simulink model "allmodes"  (Simulink 7.4)
settings: Solver=ode23tb  StartTime=0.0  StopTime=inf  MaxStep=1e-4  RelTol=1e-4
undefined symbols (not defined in the file): Ion, Lithium
libraries: powerlib x185, electricdrivelib x21, powerlib_extras x19, simulink x5
(part 3 of 7)

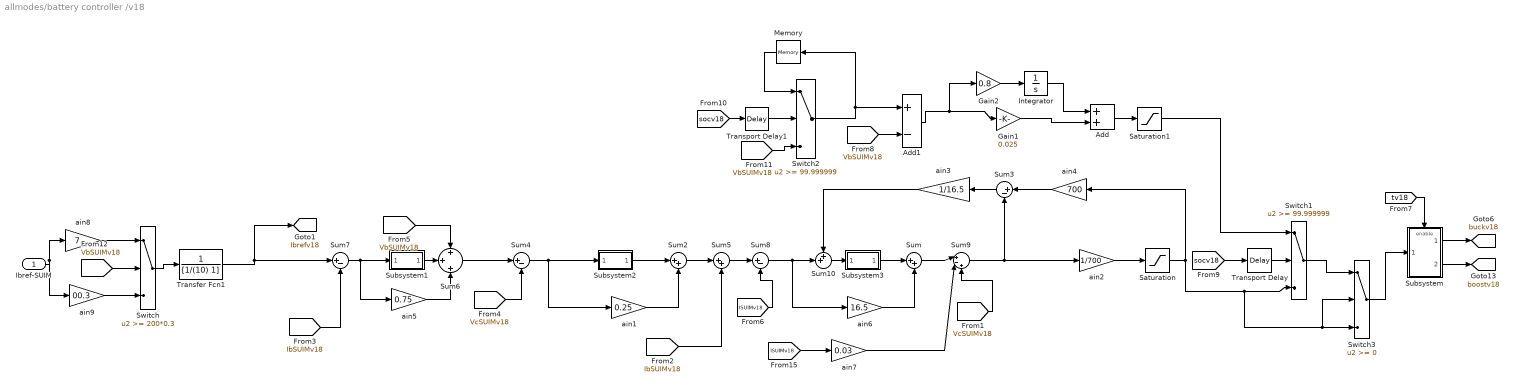
== system allmodes/battery controller /v18 ==
  Ibref-SUIM : Inport
  Add : Sum  OutDataType=fixdt(1, 16)  OutScaling=2^-10
  Add1 : Sum  Inputs=+-  OutDataType=fixdt(1, 16)  OutScaling=2^-10
  Gain1 : Gain  Gain=0.025  ParameterDataType=fixdt(1, 16)  ParameterScaling=2^0  OutDataType=fixdt(1, 16)  OutScaling=2^0
  Gain2 : Gain  Gain=0.8  ParameterDataType=fixdt(1, 16)  ParameterScaling=2^0  OutDataType=fixdt(1, 16)  OutScaling=2^0
  Integrator : Integrator
  Memory : Memory  X0=200
  Saturation : Saturate  UpperLimit=1  LowerLimit=-1  OutDataType=fixdt(1, 16)  OutScaling=2^0
  Saturation1 : Saturate  UpperLimit=1.01  LowerLimit=0.1  OutDataType=fixdt(1, 16)  OutScaling=2^0
  Subsystem : Subsystem
  Subsystem1 : Subsystem
  Subsystem2 : Subsystem
  Subsystem3 : Subsystem
  Sum : Sum  Inputs=|++  OutDataType=fixdt(1, 16)  OutScaling=2^0
  Sum10 : Sum  Inputs=++|  OutDataType=fixdt(1, 16)  OutScaling=2^0
  Sum2 : Sum  Inputs=|++  OutDataType=fixdt(1, 16)  OutScaling=2^0
  Sum{3..4,7..8} (4 alike) : Sum  Inputs=|+-  OutDataType=fixdt(1, 16)  OutScaling=2^0
  Sum5 : Sum  Inputs=|++  OutDataType=fixdt(1, 16)  OutScaling=2^0
  Sum6 : Sum  Inputs=+|+|+  OutDataType=fixdt(1, 16)  OutScaling=2^0
  Sum9 : Sum  Inputs=|+-+  OutDataType=fixdt(1, 16)  OutScaling=2^0
  Switch : Switch  Threshold=200*0.3  OutDataType=fixdt(1, 16)  OutScaling=2^0
  Switch1 : Switch  Threshold=99.999999  OutDataType=fixdt(1, 16)  OutScaling=2^0
  Switch2 : Switch  Threshold=99.999999  OutDataType=fixdt(1, 16)  OutScaling=2^0
  Switch3 : Switch  OutDataType=fixdt(1, 16)  OutScaling=2^0
  Transfer Fcn1 : TransferFcn  Numerator=1  Denominator=[1/(10) 1]
  Transport Delay : TransportDelay  DelayTime=2
  Transport Delay1 : TransportDelay  DelayTime=2
  ain1 : Gain  Gain=0.25  ParameterDataType=fixdt(1, 16)  ParameterScaling=2^0  OutDataType=fixdt(1, 16)  OutScaling=2^0
  ain2 : Gain  Gain=1/700  ParameterDataType=fixdt(1, 16)  ParameterScaling=2^0  OutDataType=fixdt(1, 16)  OutScaling=2^0
  ain3 : Gain  Gain=1/16.5  ParameterDataType=fixdt(1, 16)  ParameterScaling=2^0  OutDataType=fixdt(1, 16)  OutScaling=2^0
  ain4 : Gain  Gain=700  ParameterDataType=fixdt(1, 16)  ParameterScaling=2^0  OutDataType=fixdt(1, 16)  OutScaling=2^0
  ain5 : Gain  Gain=0.75  ParameterDataType=fixdt(1, 16)  ParameterScaling=2^0  OutDataType=fixdt(1, 16)  OutScaling=2^0
  ain6 : Gain  Gain=16.5  ParameterDataType=fixdt(1, 16)  ParameterScaling=2^0  OutDataType=fixdt(1, 16)  OutScaling=2^0
  ain7 : Gain  Gain=0.03  ParameterDataType=fixdt(1, 16)  ParameterScaling=2^0  OutDataType=fixdt(1, 16)  OutScaling=2^0
  ain8 : Gain  Gain=7  ParameterDataType=fixdt(1, 16)  ParameterScaling=2^0  OutDataType=fixdt(1, 16)  OutScaling=2^0
  ain9 : Gain  Gain=00.3  ParameterDataType=fixdt(1, 16)  ParameterScaling=2^0  OutDataType=fixdt(1, 16)  OutScaling=2^0
  tag scope: Ibrefv18=global, boostv18=global, buckv18=global
  wires:
  Ibref-SUIM/1 -> ain9/1, ain8/1
  Switch/1 -> Transfer Fcn1/1
  ain9/1 -> Switch/3
  ain8/1 -> Switch/1
  [VbSUIMv18] -> Switch/2
  Saturation1/1 -> Switch1/1
  Transport Delay/1 -> Switch1/2
  [socv18] -> Transport Delay/1
  Memory/1 -> Switch2/1
  Switch2/1 -> Memory/1, Add1/1
  Gain2/1 -> Integrator/1
  Integrator/1 -> Add/1
  Gain1/1 -> Add/2
  Add/1 -> Saturation1/1
  Transport Delay1/1 -> Switch2/2
  [socv18] -> Transport Delay1/1
  [VbSUIMv18] -> Switch2/3
  Add1/1 -> Gain2/1, Gain1/1
  [VbSUIMv18] -> Add1/2
  [tv18] -> Subsystem/Enable
  Sum4/1 -> ain1/1, Subsystem2/1(In1)
  ain2/1 -> Saturation/1
  Subsystem2/1(Out1) -> Sum2/1
  ain1/1 -> Sum2/2
  Saturation/1 -> ain4/1, Switch1/3, Switch3/3, Switch3/2
  ain4/1 -> Sum3/1
  Sum3/1 -> ain3/1
  Subsystem1/1(Out1) -> Sum6/2
  ain5/1 -> Sum6/3
  Sum7/1 -> ain5/1, Subsystem1/1(In1)
  Sum2/1 -> Sum5/1
  Sum5/1 -> Sum8/1
  Sum8/1 -> ain6/1, Sum10/2
  Subsystem3/1(Out1) -> Sum/1
  ain6/1 -> Sum/2
  Sum/1 -> Sum9/1
  Sum9/1 -> Sum3/2, ain2/1
  ain3/1 -> Sum10/1
  ain7/1 -> Sum9/2
  Sum6/1 -> Sum4/1
  Sum10/1 -> Subsystem3/1(In1)
  [VcSUIMv18] -> Sum4/2
  [VcSUIMv18] -> Sum9/3
  [IbSUIMv18] -> Sum7/2
  [IbSUIMv18] -> Sum5/2
  [VbSUIMv18] -> Sum6/1
  [ISUIMv18] -> ain7/1
  [ISUIMv18] -> Sum8/2
  Subsystem/2(Out2) -> [boostv18]
  Subsystem/1(Out1) -> [buckv18]
  Transfer Fcn1/1 -> [Ibrefv18], Sum7/1
  Switch1/1 -> Switch3/1
  Switch3/1 -> Subsystem/1(In1)

== system allmodes/battery controller /v19 ==
  Ibref-SUIM : Inport
  Add : Sum  OutDataType=fixdt(1, 16)  OutScaling=2^-10
  Add1 : Sum  Inputs=+-  OutDataType=fixdt(1, 16)  OutScaling=2^-10
  Gain1 : Gain  Gain=0.025  ParameterDataType=fixdt(1, 16)  ParameterScaling=2^0  OutDataType=fixdt(1, 16)  OutScaling=2^0
  Gain2 : Gain  Gain=0.8  ParameterDataType=fixdt(1, 16)  ParameterScaling=2^0  OutDataType=fixdt(1, 16)  OutScaling=2^0
  Integrator : Integrator
  Memory : Memory  X0=200
  Saturation : Saturate  UpperLimit=1  LowerLimit=-1  OutDataType=fixdt(1, 16)  OutScaling=2^0
  Saturation1 : Saturate  UpperLimit=1.01  LowerLimit=0.1  OutDataType=fixdt(1, 16)  OutScaling=2^0
  Subsystem : Subsystem
  Subsystem1 : Subsystem
  Subsystem2 : Subsystem
  Subsystem3 : Subsystem
  Sum : Sum  Inputs=|++  OutDataType=fixdt(1, 16)  OutScaling=2^0
  Sum10 : Sum  Inputs=++|  OutDataType=fixdt(1, 16)  OutScaling=2^0
  Sum2 : Sum  Inputs=|++  OutDataType=fixdt(1, 16)  OutScaling=2^0
  Sum{3..4,7..8} (4 alike) : Sum  Inputs=|+-  OutDataType=fixdt(1, 16)  OutScaling=2^0
  Sum5 : Sum  Inputs=|++  OutDataType=fixdt(1, 16)  OutScaling=2^0
  Sum6 : Sum  Inputs=+|+|+  OutDataType=fixdt(1, 16)  OutScaling=2^0
  Sum9 : Sum  Inputs=|+-+  OutDataType=fixdt(1, 16)  OutScaling=2^0
  Switch : Switch  Threshold=200*0.3  OutDataType=fixdt(1, 16)  OutScaling=2^0
  Switch1 : Switch  Threshold=99.999999  OutDataType=fixdt(1, 16)  OutScaling=2^0
  Switch2 : Switch  Threshold=99.999999  OutDataType=fixdt(1, 16)  OutScaling=2^0
  Switch3 : Switch  OutDataType=fixdt(1, 16)  OutScaling=2^0
  Transfer Fcn1 : TransferFcn  Numerator=1  Denominator=[1/(10) 1]
  Transport Delay : TransportDelay  DelayTime=2
  Transport Delay1 : TransportDelay  DelayTime=2
  ain1 : Gain  Gain=0.25  ParameterDataType=fixdt(1, 16)  ParameterScaling=2^0  OutDataType=fixdt(1, 16)  OutScaling=2^0
  ain2 : Gain  Gain=1/700  ParameterDataType=fixdt(1, 16)  ParameterScaling=2^0  OutDataType=fixdt(1, 16)  OutScaling=2^0
  ain3 : Gain  Gain=1/16.5  ParameterDataType=fixdt(1, 16)  ParameterScaling=2^0  OutDataType=fixdt(1, 16)  OutScaling=2^0
  ain4 : Gain  Gain=700  ParameterDataType=fixdt(1, 16)  ParameterScaling=2^0  OutDataType=fixdt(1, 16)  OutScaling=2^0
  ain5 : Gain  Gain=0.75  ParameterDataType=fixdt(1, 16)  ParameterScaling=2^0  OutDataType=fixdt(1, 16)  OutScaling=2^0
  ain6 : Gain  Gain=16.5  ParameterDataType=fixdt(1, 16)  ParameterScaling=2^0  OutDataType=fixdt(1, 16)  OutScaling=2^0
  ain7 : Gain  Gain=0.03  ParameterDataType=fixdt(1, 16)  ParameterScaling=2^0  OutDataType=fixdt(1, 16)  OutScaling=2^0
  ain8 : Gain  Gain=7  ParameterDataType=fixdt(1, 16)  ParameterScaling=2^0  OutDataType=fixdt(1, 16)  OutScaling=2^0
  ain9 : Gain  Gain=0.3  ParameterDataType=fixdt(1, 16)  ParameterScaling=2^0  OutDataType=fixdt(1, 16)  OutScaling=2^0
  tag scope: Ibrefv19=global, boostv19=global, buckv19=global
  wires:
  Ibref-SUIM/1 -> ain9/1, ain8/1
  Switch/1 -> Transfer Fcn1/1
  ain9/1 -> Switch/3
  ain8/1 -> Switch/1
  [VbSUIMv19] -> Switch/2
  Saturation1/1 -> Switch1/1
  Transport Delay/1 -> Switch1/2
  [socv19] -> Transport Delay/1
  Memory/1 -> Switch2/1
  Switch2/1 -> Memory/1, Add1/1
  Gain2/1 -> Integrator/1
  Integrator/1 -> Add/1
  Gain1/1 -> Add/2
  Add/1 -> Saturation1/1
  Transport Delay1/1 -> Switch2/2
  [socv19] -> Transport Delay1/1
  [VbSUIMv19] -> Switch2/3
  Add1/1 -> Gain2/1, Gain1/1
  [VbSUIMv19] -> Add1/2
  [tv19] -> Subsystem/Enable
  Sum4/1 -> ain1/1, Subsystem2/1(In1)
  ain2/1 -> Saturation/1
  Subsystem2/1(Out1) -> Sum2/1
  ain1/1 -> Sum2/2
  Saturation/1 -> ain4/1, Switch1/3, Switch3/3, Switch3/2
  ain4/1 -> Sum3/1
  Sum3/1 -> ain3/1
  Subsystem1/1(Out1) -> Sum6/2
  ain5/1 -> Sum6/3
  Sum7/1 -> ain5/1, Subsystem1/1(In1)
  Sum2/1 -> Sum5/1
  Sum5/1 -> Sum8/1
  Sum8/1 -> ain6/1, Sum10/2
  Subsystem3/1(Out1) -> Sum/1
  ain6/1 -> Sum/2
  Sum/1 -> Sum9/1
  Sum9/1 -> Sum3/2, ain2/1
  ain3/1 -> Sum10/1
  ain7/1 -> Sum9/2
  Sum6/1 -> Sum4/1
  Sum10/1 -> Subsystem3/1(In1)
  [VcSUIMv19] -> Sum4/2
  [VcSUIMv19] -> Sum9/3
  [IbSUIMv19] -> Sum7/2
  [IbSUIMv19] -> Sum5/2
  [VbSUIMv19] -> Sum6/1
  [ISUIMv19] -> ain7/1
  [ISUIMv19] -> Sum8/2
  Subsystem/2(Out2) -> [boostv19]
  Subsystem/1(Out1) -> [buckv19]
  Transfer Fcn1/1 -> [Ibrefv19], Sum7/1
  Switch1/1 -> Switch3/1
  Switch3/1 -> Subsystem/1(In1)

== system allmodes/battery controller /v2 ==
  Ibref-v2 : Inport
  Add : Sum  OutDataType=fixdt(1, 16)  OutScaling=2^-10
  Add1 : Sum  Inputs=+-  OutDataType=fixdt(1, 16)  OutScaling=2^-10
  Gain1 : Gain  Gain=0.025  ParameterDataType=fixdt(1, 16)  ParameterScaling=2^0  OutDataType=fixdt(1, 16)  OutScaling=2^0
  Gain2 : Gain  Gain=0.8  ParameterDataType=fixdt(1, 16)  ParameterScaling=2^0  OutDataType=fixdt(1, 16)  OutScaling=2^0
  Integrator : Integrator
  Memory : Memory  X0=200
  Saturation : Saturate  UpperLimit=1  LowerLimit=-1  OutDataType=fixdt(1, 16)  OutScaling=2^0
  Saturation1 : Saturate  UpperLimit=1.01  LowerLimit=0.1  OutDataType=fixdt(1, 16)  OutScaling=2^0
  Subsystem : Subsystem
  Subsystem1 : Subsystem
  Subsystem2 : Subsystem
  Subsystem3 : Subsystem
  Sum : Sum  Inputs=|++  OutDataType=fixdt(1, 16)  OutScaling=2^0
  Sum10 : Sum  Inputs=++|  OutDataType=fixdt(1, 16)  OutScaling=2^0
  Sum2 : Sum  Inputs=|++  OutDataType=fixdt(1, 16)  OutScaling=2^0
  Sum{3..4,7..8} (4 alike) : Sum  Inputs=|+-  OutDataType=fixdt(1, 16)  OutScaling=2^0
  Sum5 : Sum  Inputs=|++  OutDataType=fixdt(1, 16)  OutScaling=2^0
  Sum6 : Sum  Inputs=+|+|+  OutDataType=fixdt(1, 16)  OutScaling=2^0
  Sum9 : Sum  Inputs=|+-+  OutDataType=fixdt(1, 16)  OutScaling=2^0
  Switch : Switch  Threshold=200*0.3  OutDataType=fixdt(1, 16)  OutScaling=2^0
  Switch1 : Switch  Threshold=99.999999  OutDataType=fixdt(1, 16)  OutScaling=2^0
  Switch2 : Switch  Threshold=99.999999  OutDataType=fixdt(1, 16)  OutScaling=2^0
  Switch3 : Switch  OutDataType=fixdt(1, 16)  OutScaling=2^0
  Transfer Fcn1 : TransferFcn  Numerator=1  Denominator=[1/(10) 1]
  Transport Delay : TransportDelay  DelayTime=2
  Transport Delay1 : TransportDelay  DelayTime=2
  ain1 : Gain  Gain=0.25  ParameterDataType=fixdt(1, 16)  ParameterScaling=2^0  OutDataType=fixdt(1, 16)  OutScaling=2^0
  ain2 : Gain  Gain=1/700  ParameterDataType=fixdt(1, 16)  ParameterScaling=2^0  OutDataType=fixdt(1, 16)  OutScaling=2^0
  ain3 : Gain  Gain=1/16.5  ParameterDataType=fixdt(1, 16)  ParameterScaling=2^0  OutDataType=fixdt(1, 16)  OutScaling=2^0
  ain4 : Gain  Gain=700  ParameterDataType=fixdt(1, 16)  ParameterScaling=2^0  OutDataType=fixdt(1, 16)  OutScaling=2^0
  ain5 : Gain  Gain=0.75  ParameterDataType=fixdt(1, 16)  ParameterScaling=2^0  OutDataType=fixdt(1, 16)  OutScaling=2^0
  ain6 : Gain  Gain=16.5  ParameterDataType=fixdt(1, 16)  ParameterScaling=2^0  OutDataType=fixdt(1, 16)  OutScaling=2^0
  ain7 : Gain  Gain=0.03  ParameterDataType=fixdt(1, 16)  ParameterScaling=2^0  OutDataType=fixdt(1, 16)  OutScaling=2^0
  ain8 : Gain  Gain=7  ParameterDataType=fixdt(1, 16)  ParameterScaling=2^0  OutDataType=fixdt(1, 16)  OutScaling=2^0
  ain9 : Gain  Gain=0.3  ParameterDataType=fixdt(1, 16)  ParameterScaling=2^0  OutDataType=fixdt(1, 16)  OutScaling=2^0
  tag scope: Ibrefv2=global, boostv2=global, buckv2=global
  wires:
  Sum4/1 -> ain1/1, Subsystem2/1(In1)
  ain2/1 -> Saturation/1
  Subsystem2/1(Out1) -> Sum2/1
  ain1/1 -> Sum2/2
  Saturation/1 -> ain4/1, Switch1/3, Switch3/2, Switch3/3
  ain4/1 -> Sum3/1
  Sum3/1 -> ain3/1
  Subsystem1/1(Out1) -> Sum6/2
  ain5/1 -> Sum6/3
  Sum7/1 -> ain5/1, Subsystem1/1(In1)
  Sum2/1 -> Sum5/1
  Sum5/1 -> Sum8/1
  Sum8/1 -> ain6/1, Sum10/2
  Subsystem3/1(Out1) -> Sum/1
  ain6/1 -> Sum/2
  Sum/1 -> Sum9/1
  Sum9/1 -> Sum3/2, ain2/1
  ain3/1 -> Sum10/1
  ain7/1 -> Sum9/2
  Sum6/1 -> Sum4/1
  Sum10/1 -> Subsystem3/1(In1)
  [VcSUIMv2] -> Sum4/2
  [VcSUIMv2] -> Sum9/3
  [IbSUIMv2] -> Sum7/2
  [IbSUIMv2] -> Sum5/2
  [VbSUIMv2] -> Sum6/1
  [ISUIMv2] -> ain7/1
  [ISUIMv2] -> Sum8/2
  Subsystem/2(Out2) -> [boostv2]
  Subsystem/1(Out1) -> [buckv2]
  Transfer Fcn1/1 -> [Ibrefv2], Sum7/1
  [tv2] -> Subsystem/Enable
  [VbSUIMv2] -> Switch/2
  ain8/1 -> Switch/1
  ain9/1 -> Switch/3
  Ibref-v2/1 -> ain8/1, ain9/1
  Switch/1 -> Transfer Fcn1/1
  [VbSUIMv2] -> Add1/2
  Add1/1 -> Gain1/1, Gain2/1
  [VbSUIMv2] -> Switch2/3
  [socv2] -> Transport Delay1/1
  Transport Delay1/1 -> Switch2/2
  Add/1 -> Saturation1/1
  Gain1/1 -> Add/2
  Integrator/1 -> Add/1
  Gain2/1 -> Integrator/1
  Switch2/1 -> Add1/1, Memory/1
  Memory/1 -> Switch2/1
  Saturation1/1 -> Switch1/1
  Transport Delay/1 -> Switch1/2
  [socv2] -> Transport Delay/1
  Switch1/1 -> Switch3/1
  Switch3/1 -> Subsystem/1(In1)

== system allmodes/battery controller /v20 ==
  Ibref-v2 : Inport
  Add : Sum  OutDataType=fixdt(1, 16)  OutScaling=2^-10
  Add1 : Sum  Inputs=+-  OutDataType=fixdt(1, 16)  OutScaling=2^-10
  Gain1 : Gain  Gain=0.025  ParameterDataType=fixdt(1, 16)  ParameterScaling=2^0  OutDataType=fixdt(1, 16)  OutScaling=2^0
  Gain2 : Gain  Gain=0.8  ParameterDataType=fixdt(1, 16)  ParameterScaling=2^0  OutDataType=fixdt(1, 16)  OutScaling=2^0
  Integrator : Integrator
  Memory : Memory  X0=200
  Saturation : Saturate  UpperLimit=1  LowerLimit=-1  OutDataType=fixdt(1, 16)  OutScaling=2^0
  Saturation1 : Saturate  UpperLimit=1.01  LowerLimit=0.1  OutDataType=fixdt(1, 16)  OutScaling=2^0
  Subsystem : Subsystem
  Subsystem1 : Subsystem
  Subsystem2 : Subsystem
  Subsystem3 : Subsystem
  Sum : Sum  Inputs=|++  OutDataType=fixdt(1, 16)  OutScaling=2^0
  Sum10 : Sum  Inputs=++|  OutDataType=fixdt(1, 16)  OutScaling=2^0
  Sum2 : Sum  Inputs=|++  OutDataType=fixdt(1, 16)  OutScaling=2^0
  Sum{3..4,7..8} (4 alike) : Sum  Inputs=|+-  OutDataType=fixdt(1, 16)  OutScaling=2^0
  Sum5 : Sum  Inputs=|++  OutDataType=fixdt(1, 16)  OutScaling=2^0
  Sum6 : Sum  Inputs=+|+|+  OutDataType=fixdt(1, 16)  OutScaling=2^0
  Sum9 : Sum  Inputs=|+-+  OutDataType=fixdt(1, 16)  OutScaling=2^0
  Switch : Switch  Threshold=200*0.3  OutDataType=fixdt(1, 16)  OutScaling=2^0
  Switch1 : Switch  Threshold=99.999999  OutDataType=fixdt(1, 16)  OutScaling=2^0
  Switch2 : Switch  Threshold=99.999999  OutDataType=fixdt(1, 16)  OutScaling=2^0
  Switch3 : Switch  OutDataType=fixdt(1, 16)  OutScaling=2^0
  Transfer Fcn1 : TransferFcn  Numerator=1  Denominator=[1/(10) 1]
  Transport Delay : TransportDelay  DelayTime=2
  Transport Delay1 : TransportDelay  DelayTime=2
  ain1 : Gain  Gain=0.25  ParameterDataType=fixdt(1, 16)  ParameterScaling=2^0  OutDataType=fixdt(1, 16)  OutScaling=2^0
  ain2 : Gain  Gain=1/700  ParameterDataType=fixdt(1, 16)  ParameterScaling=2^0  OutDataType=fixdt(1, 16)  OutScaling=2^0
  ain3 : Gain  Gain=1/16.5  ParameterDataType=fixdt(1, 16)  ParameterScaling=2^0  OutDataType=fixdt(1, 16)  OutScaling=2^0
  ain4 : Gain  Gain=700  ParameterDataType=fixdt(1, 16)  ParameterScaling=2^0  OutDataType=fixdt(1, 16)  OutScaling=2^0
  ain5 : Gain  Gain=0.75  ParameterDataType=fixdt(1, 16)  ParameterScaling=2^0  OutDataType=fixdt(1, 16)  OutScaling=2^0
  ain6 : Gain  Gain=16.5  ParameterDataType=fixdt(1, 16)  ParameterScaling=2^0  OutDataType=fixdt(1, 16)  OutScaling=2^0
  ain7 : Gain  Gain=0.03  ParameterDataType=fixdt(1, 16)  ParameterScaling=2^0  OutDataType=fixdt(1, 16)  OutScaling=2^0
  ain8 : Gain  Gain=7  ParameterDataType=fixdt(1, 16)  ParameterScaling=2^0  OutDataType=fixdt(1, 16)  OutScaling=2^0
  ain9 : Gain  Gain=0.3  ParameterDataType=fixdt(1, 16)  ParameterScaling=2^0  OutDataType=fixdt(1, 16)  OutScaling=2^0
  tag scope: Ibrefv20=global, boostv20=global, buckv20=global
  wires:
  [socv20] -> Transport Delay/1
  Transport Delay/1 -> Switch1/2
  Saturation1/1 -> Switch1/1
  Memory/1 -> Switch2/1
  Switch2/1 -> Memory/1, Add1/1
  Gain2/1 -> Integrator/1
  Integrator/1 -> Add/1
  Gain1/1 -> Add/2
  Add/1 -> Saturation1/1
  Transport Delay1/1 -> Switch2/2
  [socv20] -> Transport Delay1/1
  [VbSUIMv20] -> Switch2/3
  Add1/1 -> Gain2/1, Gain1/1
  [VbSUIMv20] -> Add1/2
  Switch/1 -> Transfer Fcn1/1
  Ibref-v2/1 -> ain9/1, ain8/1
  ain9/1 -> Switch/3
  ain8/1 -> Switch/1
  [VbSUIMv20] -> Switch/2
  [tv20] -> Subsystem/Enable
  Transfer Fcn1/1 -> Sum7/1, [Ibrefv20]
  Subsystem/1(Out1) -> [buckv20]
  Subsystem/2(Out2) -> [boostv20]
  [ISUIMv20] -> Sum8/2
  [ISUIMv20] -> ain7/1
  [VbSUIMv20] -> Sum6/1
  [IbSUIMv20] -> Sum5/2
  [IbSUIMv20] -> Sum7/2
  [VcSUIMv20] -> Sum9/3
  [VcSUIMv20] -> Sum4/2
  Sum10/1 -> Subsystem3/1(In1)
  Sum6/1 -> Sum4/1
  ain7/1 -> Sum9/2
  ain3/1 -> Sum10/1
  Sum9/1 -> ain2/1, Sum3/2
  Sum/1 -> Sum9/1
  ain6/1 -> Sum/2
  Subsystem3/1(Out1) -> Sum/1
  Sum8/1 -> Sum10/2, ain6/1
  Sum5/1 -> Sum8/1
  Sum2/1 -> Sum5/1
  Sum7/1 -> Subsystem1/1(In1), ain5/1
  ain5/1 -> Sum6/3
  Subsystem1/1(Out1) -> Sum6/2
  Sum3/1 -> ain3/1
  ain4/1 -> Sum3/1
  Saturation/1 -> ain4/1, Switch1/3, Switch3/3, Switch3/2
  ain1/1 -> Sum2/2
  Subsystem2/1(Out1) -> Sum2/1
  ain2/1 -> Saturation/1
  Sum4/1 -> Subsystem2/1(In1), ain1/1
  Switch1/1 -> Switch3/1
  Switch3/1 -> Subsystem/1(In1)

== system allmodes/battery controller /v3 ==
  Ibref-v2 : Inport
  Add : Sum  OutDataType=fixdt(1, 16)  OutScaling=2^-10
  Add1 : Sum  Inputs=+-  OutDataType=fixdt(1, 16)  OutScaling=2^-10
  Gain1 : Gain  Gain=0.025  ParameterDataType=fixdt(1, 16)  ParameterScaling=2^0  OutDataType=fixdt(1, 16)  OutScaling=2^0
  Gain2 : Gain  Gain=0.8  ParameterDataType=fixdt(1, 16)  ParameterScaling=2^0  OutDataType=fixdt(1, 16)  OutScaling=2^0
  Integrator : Integrator
  Memory : Memory  X0=200
  Saturation : Saturate  UpperLimit=1  LowerLimit=-1  OutDataType=fixdt(1, 16)  OutScaling=2^0
  Saturation1 : Saturate  UpperLimit=1.01  LowerLimit=0.1  OutDataType=fixdt(1, 16)  OutScaling=2^0
  Subsystem : Subsystem
  Subsystem1 : Subsystem
  Subsystem2 : Subsystem
  Subsystem3 : Subsystem
  Sum : Sum  Inputs=|++  OutDataType=fixdt(1, 16)  OutScaling=2^0
  Sum10 : Sum  Inputs=++|  OutDataType=fixdt(1, 16)  OutScaling=2^0
  Sum2 : Sum  Inputs=|++  OutDataType=fixdt(1, 16)  OutScaling=2^0
  Sum{3..4,7..8} (4 alike) : Sum  Inputs=|+-  OutDataType=fixdt(1, 16)  OutScaling=2^0
  Sum5 : Sum  Inputs=|++  OutDataType=fixdt(1, 16)  OutScaling=2^0
  Sum6 : Sum  Inputs=+|+|+  OutDataType=fixdt(1, 16)  OutScaling=2^0
  Sum9 : Sum  Inputs=|+-+  OutDataType=fixdt(1, 16)  OutScaling=2^0
  Switch : Switch  Threshold=200*0.3  OutDataType=fixdt(1, 16)  OutScaling=2^0
  Switch1 : Switch  Threshold=99.999999  OutDataType=fixdt(1, 16)  OutScaling=2^0
  Switch2 : Switch  Threshold=99.999999  OutDataType=fixdt(1, 16)  OutScaling=2^0
  Switch3 : Switch  OutDataType=fixdt(1, 16)  OutScaling=2^0
  Transfer Fcn1 : TransferFcn  Numerator=1  Denominator=[1/(10) 1]
  Transport Delay : TransportDelay  DelayTime=2
  Transport Delay1 : TransportDelay  DelayTime=2
  ain1 : Gain  Gain=0.25  ParameterDataType=fixdt(1, 16)  ParameterScaling=2^0  OutDataType=fixdt(1, 16)  OutScaling=2^0
  ain2 : Gain  Gain=1/700  ParameterDataType=fixdt(1, 16)  ParameterScaling=2^0  OutDataType=fixdt(1, 16)  OutScaling=2^0
  ain3 : Gain  Gain=1/16.5  ParameterDataType=fixdt(1, 16)  ParameterScaling=2^0  OutDataType=fixdt(1, 16)  OutScaling=2^0
  ain4 : Gain  Gain=700  ParameterDataType=fixdt(1, 16)  ParameterScaling=2^0  OutDataType=fixdt(1, 16)  OutScaling=2^0
  ain5 : Gain  Gain=0.75  ParameterDataType=fixdt(1, 16)  ParameterScaling=2^0  OutDataType=fixdt(1, 16)  OutScaling=2^0
  ain6 : Gain  Gain=16.5  ParameterDataType=fixdt(1, 16)  ParameterScaling=2^0  OutDataType=fixdt(1, 16)  OutScaling=2^0
  ain7 : Gain  Gain=0.03  ParameterDataType=fixdt(1, 16)  ParameterScaling=2^0  OutDataType=fixdt(1, 16)  OutScaling=2^0
  ain8 : Gain  Gain=7  ParameterDataType=fixdt(1, 16)  ParameterScaling=2^0  OutDataType=fixdt(1, 16)  OutScaling=2^0
  ain9 : Gain  Gain=0.3  ParameterDataType=fixdt(1, 16)  ParameterScaling=2^0  OutDataType=fixdt(1, 16)  OutScaling=2^0
  tag scope: Ibrefv3=global, boostv3=global, buckv3=global
  wires:
  [socv3] -> Transport Delay/1
  Transport Delay/1 -> Switch1/2
  Saturation1/1 -> Switch1/1
  Memory/1 -> Switch2/1
  Switch2/1 -> Memory/1, Add1/1
  Gain2/1 -> Integrator/1
  Integrator/1 -> Add/1
  Gain1/1 -> Add/2
  Add/1 -> Saturation1/1
  Transport Delay1/1 -> Switch2/2
  [socv3] -> Transport Delay1/1
  [VbSUIMv3] -> Switch2/3
  Add1/1 -> Gain2/1, Gain1/1
  [VbSUIMv3] -> Add1/2
  Switch/1 -> Transfer Fcn1/1
  Ibref-v2/1 -> ain9/1, ain8/1
  ain9/1 -> Switch/3
  ain8/1 -> Switch/1
  [VbSUIMv3] -> Switch/2
  [tv3] -> Subsystem/Enable
  Transfer Fcn1/1 -> Sum7/1, [Ibrefv3]
  Subsystem/1(Out1) -> [buckv3]
  Subsystem/2(Out2) -> [boostv3]
  [ISUIMv3] -> Sum8/2
  [ISUIMv3] -> ain7/1
  [VbSUIMv3] -> Sum6/1
  [IbSUIMv3] -> Sum5/2
  [IbSUIMv3] -> Sum7/2
  [VcSUIMv3] -> Sum9/3
  [VcSUIMv3] -> Sum4/2
  Sum10/1 -> Subsystem3/1(In1)
  Sum6/1 -> Sum4/1
  ain7/1 -> Sum9/2
  ain3/1 -> Sum10/1
  Sum9/1 -> ain2/1, Sum3/2
  Sum/1 -> Sum9/1
  ain6/1 -> Sum/2
  Subsystem3/1(Out1) -> Sum/1
  Sum8/1 -> Sum10/2, ain6/1
  Sum5/1 -> Sum8/1
  Sum2/1 -> Sum5/1
  Sum7/1 -> Subsystem1/1(In1), ain5/1
  ain5/1 -> Sum6/3
  Subsystem1/1(Out1) -> Sum6/2
  Sum3/1 -> ain3/1
  ain4/1 -> Sum3/1
  Saturation/1 -> ain4/1, Switch1/3, Switch3/2, Switch3/3
  ain1/1 -> Sum2/2
  Subsystem2/1(Out1) -> Sum2/1
  ain2/1 -> Saturation/1
  Sum4/1 -> Subsystem2/1(In1), ain1/1
  Switch1/1 -> Switch3/1
  Switch3/1 -> Subsystem/1(In1)

== system allmodes/battery controller /v4 ==
  Ibref-v2 : Inport
  Add : Sum  OutDataType=fixdt(1, 16)  OutScaling=2^-10
  Add1 : Sum  Inputs=+-  OutDataType=fixdt(1, 16)  OutScaling=2^-10
  Gain1 : Gain  Gain=0.025  ParameterDataType=fixdt(1, 16)  ParameterScaling=2^0  OutDataType=fixdt(1, 16)  OutScaling=2^0
  Gain2 : Gain  Gain=0.8  ParameterDataType=fixdt(1, 16)  ParameterScaling=2^0  OutDataType=fixdt(1, 16)  OutScaling=2^0
  Integrator : Integrator
  Memory : Memory  X0=200
  Saturation : Saturate  UpperLimit=1  LowerLimit=-1  OutDataType=fixdt(1, 16)  OutScaling=2^0
  Saturation1 : Saturate  UpperLimit=1.01  LowerLimit=0.1  OutDataType=fixdt(1, 16)  OutScaling=2^0
  Subsystem : Subsystem
  Subsystem1 : Subsystem
  Subsystem2 : Subsystem
  Subsystem3 : Subsystem
  Sum : Sum  Inputs=|++  OutDataType=fixdt(1, 16)  OutScaling=2^0
  Sum10 : Sum  Inputs=++|  OutDataType=fixdt(1, 16)  OutScaling=2^0
  Sum2 : Sum  Inputs=|++  OutDataType=fixdt(1, 16)  OutScaling=2^0
  Sum{3..4,7..8} (4 alike) : Sum  Inputs=|+-  OutDataType=fixdt(1, 16)  OutScaling=2^0
  Sum5 : Sum  Inputs=|++  OutDataType=fixdt(1, 16)  OutScaling=2^0
  Sum6 : Sum  Inputs=+|+|+  OutDataType=fixdt(1, 16)  OutScaling=2^0
  Sum9 : Sum  Inputs=|+-+  OutDataType=fixdt(1, 16)  OutScaling=2^0
  Switch : Switch  Threshold=200*0.3  OutDataType=fixdt(1, 16)  OutScaling=2^0
  Switch1 : Switch  Threshold=99.999999  OutDataType=fixdt(1, 16)  OutScaling=2^0
  Switch2 : Switch  Threshold=99.999999  OutDataType=fixdt(1, 16)  OutScaling=2^0
  Switch3 : Switch  OutDataType=fixdt(1, 16)  OutScaling=2^0
  Transfer Fcn1 : TransferFcn  Numerator=1  Denominator=[1/(10) 1]
  Transport Delay : TransportDelay  DelayTime=2
  Transport Delay1 : TransportDelay  DelayTime=2
  ain1 : Gain  Gain=0.25  ParameterDataType=fixdt(1, 16)  ParameterScaling=2^0  OutDataType=fixdt(1, 16)  OutScaling=2^0
  ain2 : Gain  Gain=1/700  ParameterDataType=fixdt(1, 16)  ParameterScaling=2^0  OutDataType=fixdt(1, 16)  OutScaling=2^0
  ain3 : Gain  Gain=1/16.5  ParameterDataType=fixdt(1, 16)  ParameterScaling=2^0  OutDataType=fixdt(1, 16)  OutScaling=2^0
  ain4 : Gain  Gain=700  ParameterDataType=fixdt(1, 16)  ParameterScaling=2^0  OutDataType=fixdt(1, 16)  OutScaling=2^0
  ain5 : Gain  Gain=0.75  ParameterDataType=fixdt(1, 16)  ParameterScaling=2^0  OutDataType=fixdt(1, 16)  OutScaling=2^0
  ain6 : Gain  Gain=16.5  ParameterDataType=fixdt(1, 16)  ParameterScaling=2^0  OutDataType=fixdt(1, 16)  OutScaling=2^0
  ain7 : Gain  Gain=0.03  ParameterDataType=fixdt(1, 16)  ParameterScaling=2^0  OutDataType=fixdt(1, 16)  OutScaling=2^0
  ain8 : Gain  Gain=7  ParameterDataType=fixdt(1, 16)  ParameterScaling=2^0  OutDataType=fixdt(1, 16)  OutScaling=2^0
  ain9 : Gain  Gain=0.3  ParameterDataType=fixdt(1, 16)  ParameterScaling=2^0  OutDataType=fixdt(1, 16)  OutScaling=2^0
  tag scope: Ibrefv4=global, boostv4=global, buckv4=global
  wires:
  Sum4/1 -> ain1/1, Subsystem2/1(In1)
  ain2/1 -> Saturation/1
  Subsystem2/1(Out1) -> Sum2/1
  ain1/1 -> Sum2/2
  Saturation/1 -> ain4/1, Switch1/3, Switch3/2, Switch3/3
  ain4/1 -> Sum3/1
  Sum3/1 -> ain3/1
  Subsystem1/1(Out1) -> Sum6/2
  ain5/1 -> Sum6/3
  Sum7/1 -> ain5/1, Subsystem1/1(In1)
  Sum2/1 -> Sum5/1
  Sum5/1 -> Sum8/1
  Sum8/1 -> ain6/1, Sum10/2
  Subsystem3/1(Out1) -> Sum/1
  ain6/1 -> Sum/2
  Sum/1 -> Sum9/1
  Sum9/1 -> Sum3/2, ain2/1
  ain3/1 -> Sum10/1
  ain7/1 -> Sum9/2
  Sum6/1 -> Sum4/1
  Sum10/1 -> Subsystem3/1(In1)
  [VcSUIMv4] -> Sum4/2
  [VcSUIMv4] -> Sum9/3
  [IbSUIMv4] -> Sum7/2
  [IbSUIMv4] -> Sum5/2
  [VbSUIMv4] -> Sum6/1
  [ISUIMv4] -> ain7/1
  [ISUIMv4] -> Sum8/2
  Subsystem/2(Out2) -> [boostv4]
  Subsystem/1(Out1) -> [buckv4]
  Transfer Fcn1/1 -> [Ibrefv4], Sum7/1
  [tv4] -> Subsystem/Enable
  [VbSUIMv4] -> Switch/2
  ain8/1 -> Switch/1
  ain9/1 -> Switch/3
  Ibref-v2/1 -> ain8/1, ain9/1
  Switch/1 -> Transfer Fcn1/1
  [VbSUIMv4] -> Add1/2
  Add1/1 -> Gain1/1, Gain2/1
  [VbSUIMv4] -> Switch2/3
  [socv4] -> Transport Delay1/1
  Transport Delay1/1 -> Switch2/2
  Add/1 -> Saturation1/1
  Gain1/1 -> Add/2
  Integrator/1 -> Add/1
  Gain2/1 -> Integrator/1
  Switch2/1 -> Add1/1, Memory/1
  Memory/1 -> Switch2/1
  Saturation1/1 -> Switch1/1
  Transport Delay/1 -> Switch1/2
  [socv4] -> Transport Delay/1
  Switch1/1 -> Switch3/1
  Switch3/1 -> Subsystem/1(In1)

== system allmodes/battery controller /v5 ==
  Ibref-v2 : Inport
  Add : Sum  OutDataType=fixdt(1, 16)  OutScaling=2^-10
  Add1 : Sum  Inputs=+-  OutDataType=fixdt(1, 16)  OutScaling=2^-10
  Gain1 : Gain  Gain=0.025  ParameterDataType=fixdt(1, 16)  ParameterScaling=2^0  OutDataType=fixdt(1, 16)  OutScaling=2^0
  Gain2 : Gain  Gain=0.8  ParameterDataType=fixdt(1, 16)  ParameterScaling=2^0  OutDataType=fixdt(1, 16)  OutScaling=2^0
  Integrator : Integrator
  Memory : Memory  X0=200
  Saturation : Saturate  UpperLimit=1  LowerLimit=-1  OutDataType=fixdt(1, 16)  OutScaling=2^0
  Saturation1 : Saturate  UpperLimit=1.01  LowerLimit=0.1  OutDataType=fixdt(1, 16)  OutScaling=2^0
  Subsystem : Subsystem
  Subsystem1 : Subsystem
  Subsystem2 : Subsystem
  Subsystem3 : Subsystem
  Sum : Sum  Inputs=|++  OutDataType=fixdt(1, 16)  OutScaling=2^0
  Sum10 : Sum  Inputs=++|  OutDataType=fixdt(1, 16)  OutScaling=2^0
  Sum2 : Sum  Inputs=|++  OutDataType=fixdt(1, 16)  OutScaling=2^0
  Sum{3..4,7..8} (4 alike) : Sum  Inputs=|+-  OutDataType=fixdt(1, 16)  OutScaling=2^0
  Sum5 : Sum  Inputs=|++  OutDataType=fixdt(1, 16)  OutScaling=2^0
  Sum6 : Sum  Inputs=+|+|+  OutDataType=fixdt(1, 16)  OutScaling=2^0
  Sum9 : Sum  Inputs=|+-+  OutDataType=fixdt(1, 16)  OutScaling=2^0
  Switch : Switch  Threshold=200*0.3  OutDataType=fixdt(1, 16)  OutScaling=2^0
  Switch1 : Switch  Threshold=99.999999  OutDataType=fixdt(1, 16)  OutScaling=2^0
  Switch2 : Switch  Threshold=99.999999  OutDataType=fixdt(1, 16)  OutScaling=2^0
  Switch3 : Switch  OutDataType=fixdt(1, 16)  OutScaling=2^0
  Transfer Fcn1 : TransferFcn  Numerator=1  Denominator=[1/(10) 1]
  Transport Delay : TransportDelay  DelayTime=2
  Transport Delay1 : TransportDelay  DelayTime=2
  ain1 : Gain  Gain=0.25  ParameterDataType=fixdt(1, 16)  ParameterScaling=2^0  OutDataType=fixdt(1, 16)  OutScaling=2^0
  ain2 : Gain  Gain=1/700  ParameterDataType=fixdt(1, 16)  ParameterScaling=2^0  OutDataType=fixdt(1, 16)  OutScaling=2^0
  ain3 : Gain  Gain=1/16.5  ParameterDataType=fixdt(1, 16)  ParameterScaling=2^0  OutDataType=fixdt(1, 16)  OutScaling=2^0
  ain4 : Gain  Gain=700  ParameterDataType=fixdt(1, 16)  ParameterScaling=2^0  OutDataType=fixdt(1, 16)  OutScaling=2^0
  ain5 : Gain  Gain=0.75  ParameterDataType=fixdt(1, 16)  ParameterScaling=2^0  OutDataType=fixdt(1, 16)  OutScaling=2^0
  ain6 : Gain  Gain=16.5  ParameterDataType=fixdt(1, 16)  ParameterScaling=2^0  OutDataType=fixdt(1, 16)  OutScaling=2^0
  ain7 : Gain  Gain=0.03  ParameterDataType=fixdt(1, 16)  ParameterScaling=2^0  OutDataType=fixdt(1, 16)  OutScaling=2^0
  ain8 : Gain  Gain=7  ParameterDataType=fixdt(1, 16)  ParameterScaling=2^0  OutDataType=fixdt(1, 16)  OutScaling=2^0
  ain9 : Gain  Gain=0.3  ParameterDataType=fixdt(1, 16)  ParameterScaling=2^0  OutDataType=fixdt(1, 16)  OutScaling=2^0
  tag scope: Ibrefv5=global, boostv5=global, buckv5=global
  wires:
  [socv5] -> Transport Delay/1
  Transport Delay/1 -> Switch1/2
  Saturation1/1 -> Switch1/1
  Memory/1 -> Switch2/1
  Switch2/1 -> Memory/1, Add1/1
  Gain2/1 -> Integrator/1
  Integrator/1 -> Add/1
  Gain1/1 -> Add/2
  Add/1 -> Saturation1/1
  Transport Delay1/1 -> Switch2/2
  [socv5] -> Transport Delay1/1
  [VbSUIMv5] -> Switch2/3
  Add1/1 -> Gain2/1, Gain1/1
  [VbSUIMv5] -> Add1/2
  Switch/1 -> Transfer Fcn1/1
  Ibref-v2/1 -> ain9/1, ain8/1
  ain9/1 -> Switch/3
  ain8/1 -> Switch/1
  [VbSUIMv5] -> Switch/2
  [tv5] -> Subsystem/Enable
  Transfer Fcn1/1 -> Sum7/1, [Ibrefv5]
  Subsystem/1(Out1) -> [buckv5]
  Subsystem/2(Out2) -> [boostv5]
  [ISUIMv5] -> Sum8/2
  [ISUIMv5] -> ain7/1
  [VbSUIMv5] -> Sum6/1
  [IbSUIMv5] -> Sum5/2
  [IbSUIMv5] -> Sum7/2
  [VcSUIMv5] -> Sum9/3
  [VcSUIMv5] -> Sum4/2
  Sum10/1 -> Subsystem3/1(In1)
  Sum6/1 -> Sum4/1
  ain7/1 -> Sum9/2
  ain3/1 -> Sum10/1
  Sum9/1 -> ain2/1, Sum3/2
  Sum/1 -> Sum9/1
  ain6/1 -> Sum/2
  Subsystem3/1(Out1) -> Sum/1
  Sum8/1 -> Sum10/2, ain6/1
  Sum5/1 -> Sum8/1
  Sum2/1 -> Sum5/1
  Sum7/1 -> Subsystem1/1(In1), ain5/1
  ain5/1 -> Sum6/3
  Subsystem1/1(Out1) -> Sum6/2
  Sum3/1 -> ain3/1
  ain4/1 -> Sum3/1
  Saturation/1 -> ain4/1, Switch1/3, Switch3/3, Switch3/2
  ain1/1 -> Sum2/2
  Subsystem2/1(Out1) -> Sum2/1
  ain2/1 -> Saturation/1
  Sum4/1 -> Subsystem2/1(In1), ain1/1
  Switch1/1 -> Switch3/1
  Switch3/1 -> Subsystem/1(In1)

== system allmodes/battery controller /v6 ==
  Ibref-v2 : Inport
  Add : Sum  OutDataType=fixdt(1, 16)  OutScaling=2^-10
  Add1 : Sum  Inputs=+-  OutDataType=fixdt(1, 16)  OutScaling=2^-10
  Gain1 : Gain  Gain=0.025  ParameterDataType=fixdt(1, 16)  ParameterScaling=2^0  OutDataType=fixdt(1, 16)  OutScaling=2^0
  Gain2 : Gain  Gain=0.8  ParameterDataType=fixdt(1, 16)  ParameterScaling=2^0  OutDataType=fixdt(1, 16)  OutScaling=2^0
  Integrator : Integrator
  Memory : Memory  X0=200
  Saturation : Saturate  UpperLimit=1  LowerLimit=-1  OutDataType=fixdt(1, 16)  OutScaling=2^0
  Saturation1 : Saturate  UpperLimit=1.01  LowerLimit=0.1  OutDataType=fixdt(1, 16)  OutScaling=2^0
  Subsystem : Subsystem
  Subsystem1 : Subsystem
  Subsystem2 : Subsystem
  Subsystem3 : Subsystem
  Sum : Sum  Inputs=|++  OutDataType=fixdt(1, 16)  OutScaling=2^0
  Sum10 : Sum  Inputs=++|  OutDataType=fixdt(1, 16)  OutScaling=2^0
  Sum2 : Sum  Inputs=|++  OutDataType=fixdt(1, 16)  OutScaling=2^0
  Sum{3..4,7..8} (4 alike) : Sum  Inputs=|+-  OutDataType=fixdt(1, 16)  OutScaling=2^0
  Sum5 : Sum  Inputs=|++  OutDataType=fixdt(1, 16)  OutScaling=2^0
  Sum6 : Sum  Inputs=+|+|+  OutDataType=fixdt(1, 16)  OutScaling=2^0
  Sum9 : Sum  Inputs=|+-+  OutDataType=fixdt(1, 16)  OutScaling=2^0
  Switch : Switch  Threshold=200*0.3  OutDataType=fixdt(1, 16)  OutScaling=2^0
  Switch1 : Switch  Threshold=99.999999  OutDataType=fixdt(1, 16)  OutScaling=2^0
  Switch2 : Switch  Threshold=99.999999  OutDataType=fixdt(1, 16)  OutScaling=2^0
  Switch3 : Switch  OutDataType=fixdt(1, 16)  OutScaling=2^0
  Transfer Fcn1 : TransferFcn  Numerator=1  Denominator=[1/(10) 1]
  Transport Delay : TransportDelay  DelayTime=2
  Transport Delay1 : TransportDelay  DelayTime=2
  ain1 : Gain  Gain=0.25  ParameterDataType=fixdt(1, 16)  ParameterScaling=2^0  OutDataType=fixdt(1, 16)  OutScaling=2^0
  ain2 : Gain  Gain=1/700  ParameterDataType=fixdt(1, 16)  ParameterScaling=2^0  OutDataType=fixdt(1, 16)  OutScaling=2^0
  ain3 : Gain  Gain=1/16.5  ParameterDataType=fixdt(1, 16)  ParameterScaling=2^0  OutDataType=fixdt(1, 16)  OutScaling=2^0
  ain4 : Gain  Gain=700  ParameterDataType=fixdt(1, 16)  ParameterScaling=2^0  OutDataType=fixdt(1, 16)  OutScaling=2^0
  ain5 : Gain  Gain=0.75  ParameterDataType=fixdt(1, 16)  ParameterScaling=2^0  OutDataType=fixdt(1, 16)  OutScaling=2^0
  ain6 : Gain  Gain=16.5  ParameterDataType=fixdt(1, 16)  ParameterScaling=2^0  OutDataType=fixdt(1, 16)  OutScaling=2^0
  ain7 : Gain  Gain=0.03  ParameterDataType=fixdt(1, 16)  ParameterScaling=2^0  OutDataType=fixdt(1, 16)  OutScaling=2^0
  ain8 : Gain  Gain=7  ParameterDataType=fixdt(1, 16)  ParameterScaling=2^0  OutDataType=fixdt(1, 16)  OutScaling=2^0
  ain9 : Gain  Gain=.3  ParameterDataType=fixdt(1, 16)  ParameterScaling=2^0  OutDataType=fixdt(1, 16)  OutScaling=2^0
  tag scope: Ibrefv6=global, boostv6=global, buckv6=global
  wires:
  Sum4/1 -> ain1/1, Subsystem2/1(In1)
  ain2/1 -> Saturation/1
  Subsystem2/1(Out1) -> Sum2/1
  ain1/1 -> Sum2/2
  Saturation/1 -> ain4/1, Switch1/3, Switch3/3, Switch3/2
  ain4/1 -> Sum3/1
  Sum3/1 -> ain3/1
  Subsystem1/1(Out1) -> Sum6/2
  ain5/1 -> Sum6/3
  Sum7/1 -> ain5/1, Subsystem1/1(In1)
  Sum2/1 -> Sum5/1
  Sum5/1 -> Sum8/1
  Sum8/1 -> ain6/1, Sum10/2
  Subsystem3/1(Out1) -> Sum/1
  ain6/1 -> Sum/2
  Sum/1 -> Sum9/1
  Sum9/1 -> Sum3/2, ain2/1
  ain3/1 -> Sum10/1
  ain7/1 -> Sum9/2
  Sum6/1 -> Sum4/1
  Sum10/1 -> Subsystem3/1(In1)
  [VcSUIMv6] -> Sum4/2
  [VcSUIMv6] -> Sum9/3
  [IbSUIMv6] -> Sum7/2
  [IbSUIMv6] -> Sum5/2
  [VbSUIMv6] -> Sum6/1
  [ISUIMv6] -> ain7/1
  [ISUIMv6] -> Sum8/2
  Subsystem/2(Out2) -> [boostv6]
  Subsystem/1(Out1) -> [buckv6]
  Transfer Fcn1/1 -> [Ibrefv6], Sum7/1
  [tv6] -> Subsystem/Enable
  [VbSUIMv6] -> Switch/2
  ain8/1 -> Switch/1
  ain9/1 -> Switch/3
  Ibref-v2/1 -> ain8/1, ain9/1
  Switch/1 -> Transfer Fcn1/1
  [VbSUIMv6] -> Add1/2
  Add1/1 -> Gain1/1, Gain2/1
  [VbSUIMv6] -> Switch2/3
  [socv6] -> Transport Delay1/1
  Transport Delay1/1 -> Switch2/2
  Add/1 -> Saturation1/1
  Gain1/1 -> Add/2
  Integrator/1 -> Add/1
  Gain2/1 -> Integrator/1
  Switch2/1 -> Add1/1, Memory/1
  Memory/1 -> Switch2/1
  Saturation1/1 -> Switch1/1
  Transport Delay/1 -> Switch1/2
  [socv6] -> Transport Delay/1
  Switch1/1 -> Switch3/1
  Switch3/1 -> Subsystem/1(In1)

== system allmodes/battery controller /v7 ==
  Ibref-v2 : Inport
  Add : Sum  OutDataType=fixdt(1, 16)  OutScaling=2^-10
  Add1 : Sum  Inputs=+-  OutDataType=fixdt(1, 16)  OutScaling=2^-10
  Gain1 : Gain  Gain=0.025  ParameterDataType=fixdt(1, 16)  ParameterScaling=2^0  OutDataType=fixdt(1, 16)  OutScaling=2^0
  Gain2 : Gain  Gain=0.8  ParameterDataType=fixdt(1, 16)  ParameterScaling=2^0  OutDataType=fixdt(1, 16)  OutScaling=2^0
  Integrator : Integrator
  Memory : Memory  X0=200
  Saturation : Saturate  UpperLimit=1  LowerLimit=-1  OutDataType=fixdt(1, 16)  OutScaling=2^0
  Saturation1 : Saturate  UpperLimit=1.01  LowerLimit=0.1  OutDataType=fixdt(1, 16)  OutScaling=2^0
  Subsystem : Subsystem
  Subsystem1 : Subsystem
  Subsystem2 : Subsystem
  Subsystem3 : Subsystem
  Sum : Sum  Inputs=|++  OutDataType=fixdt(1, 16)  OutScaling=2^0
  Sum10 : Sum  Inputs=++|  OutDataType=fixdt(1, 16)  OutScaling=2^0
  Sum2 : Sum  Inputs=|++  OutDataType=fixdt(1, 16)  OutScaling=2^0
  Sum{3..4,7..8} (4 alike) : Sum  Inputs=|+-  OutDataType=fixdt(1, 16)  OutScaling=2^0
  Sum5 : Sum  Inputs=|++  OutDataType=fixdt(1, 16)  OutScaling=2^0
  Sum6 : Sum  Inputs=+|+|+  OutDataType=fixdt(1, 16)  OutScaling=2^0
  Sum9 : Sum  Inputs=|+-+  OutDataType=fixdt(1, 16)  OutScaling=2^0
  Switch : Switch  Threshold=200*0.3  OutDataType=fixdt(1, 16)  OutScaling=2^0
  Switch1 : Switch  Threshold=99.999999  OutDataType=fixdt(1, 16)  OutScaling=2^0
  Switch2 : Switch  Threshold=99.999999  OutDataType=fixdt(1, 16)  OutScaling=2^0
  Switch3 : Switch  OutDataType=fixdt(1, 16)  OutScaling=2^0
  Transfer Fcn1 : TransferFcn  Numerator=1  Denominator=[1/(10) 1]
  Transport Delay : TransportDelay  DelayTime=2
  Transport Delay1 : TransportDelay  DelayTime=2
  ain1 : Gain  Gain=0.25  ParameterDataType=fixdt(1, 16)  ParameterScaling=2^0  OutDataType=fixdt(1, 16)  OutScaling=2^0
  ain2 : Gain  Gain=1/700  ParameterDataType=fixdt(1, 16)  ParameterScaling=2^0  OutDataType=fixdt(1, 16)  OutScaling=2^0
  ain3 : Gain  Gain=1/16.5  ParameterDataType=fixdt(1, 16)  ParameterScaling=2^0  OutDataType=fixdt(1, 16)  OutScaling=2^0
  ain4 : Gain  Gain=700  ParameterDataType=fixdt(1, 16)  ParameterScaling=2^0  OutDataType=fixdt(1, 16)  OutScaling=2^0
  ain5 : Gain  Gain=0.75  ParameterDataType=fixdt(1, 16)  ParameterScaling=2^0  OutDataType=fixdt(1, 16)  OutScaling=2^0
  ain6 : Gain  Gain=16.5  ParameterDataType=fixdt(1, 16)  ParameterScaling=2^0  OutDataType=fixdt(1, 16)  OutScaling=2^0
  ain7 : Gain  Gain=0.03  ParameterDataType=fixdt(1, 16)  ParameterScaling=2^0  OutDataType=fixdt(1, 16)  OutScaling=2^0
  ain8 : Gain  Gain=7  ParameterDataType=fixdt(1, 16)  ParameterScaling=2^0  OutDataType=fixdt(1, 16)  OutScaling=2^0
  ain9 : Gain  Gain=0.3  ParameterDataType=fixdt(1, 16)  ParameterScaling=2^0  OutDataType=fixdt(1, 16)  OutScaling=2^0
  tag scope: Ibrefv7=global, boostv7=global, buckv7=global
  wires:
  [socv7] -> Transport Delay/1
  Transport Delay/1 -> Switch1/2
  Saturation1/1 -> Switch1/1
  Memory/1 -> Switch2/1
  Switch2/1 -> Memory/1, Add1/1
  Gain2/1 -> Integrator/1
  Integrator/1 -> Add/1
  Gain1/1 -> Add/2
  Add/1 -> Saturation1/1
  Transport Delay1/1 -> Switch2/2
  [socv7] -> Transport Delay1/1
  [VbSUIMv7] -> Switch2/3
  Add1/1 -> Gain2/1, Gain1/1
  [VbSUIMv7] -> Add1/2
  Switch/1 -> Transfer Fcn1/1
  Ibref-v2/1 -> ain9/1, ain8/1
  ain9/1 -> Switch/3
  ain8/1 -> Switch/1
  [VbSUIMv7] -> Switch/2
  [tv7] -> Subsystem/Enable
  Transfer Fcn1/1 -> Sum7/1, [Ibrefv7]
  Subsystem/1(Out1) -> [buckv7]
  Subsystem/2(Out2) -> [boostv7]
  [ISUIMv7] -> Sum8/2
  [ISUIMv7] -> ain7/1
  [VbSUIMv7] -> Sum6/1
  [IbSUIMv7] -> Sum5/2
  [IbSUIMv7] -> Sum7/2
  [VcSUIMv7] -> Sum9/3
  [VcSUIMv7] -> Sum4/2
  Sum10/1 -> Subsystem3/1(In1)
  Sum6/1 -> Sum4/1
  ain7/1 -> Sum9/2
  ain3/1 -> Sum10/1
  Sum9/1 -> ain2/1, Sum3/2
  Sum/1 -> Sum9/1
  ain6/1 -> Sum/2
  Subsystem3/1(Out1) -> Sum/1
  Sum8/1 -> Sum10/2, ain6/1
  Sum5/1 -> Sum8/1
  Sum2/1 -> Sum5/1
  Sum7/1 -> Subsystem1/1(In1), ain5/1
  ain5/1 -> Sum6/3
  Subsystem1/1(Out1) -> Sum6/2
  Sum3/1 -> ain3/1
  ain4/1 -> Sum3/1
  Saturation/1 -> ain4/1, Switch1/3, Switch3/3, Switch3/2
  ain1/1 -> Sum2/2
  Subsystem2/1(Out1) -> Sum2/1
  ain2/1 -> Saturation/1
  Sum4/1 -> Subsystem2/1(In1), ain1/1
  Switch1/1 -> Switch3/1
  Switch3/1 -> Subsystem/1(In1)

== system allmodes/battery controller /v8 ==
  Ibref-v2 : Inport
  Add : Sum  OutDataType=fixdt(1, 16)  OutScaling=2^-10
  Add1 : Sum  Inputs=+-  OutDataType=fixdt(1, 16)  OutScaling=2^-10
  Gain1 : Gain  Gain=0.025  ParameterDataType=fixdt(1, 16)  ParameterScaling=2^0  OutDataType=fixdt(1, 16)  OutScaling=2^0
  Gain2 : Gain  Gain=0.8  ParameterDataType=fixdt(1, 16)  ParameterScaling=2^0  OutDataType=fixdt(1, 16)  OutScaling=2^0
  Integrator : Integrator
  Memory : Memory  X0=200
  Saturation : Saturate  UpperLimit=1  LowerLimit=-1  OutDataType=fixdt(1, 16)  OutScaling=2^0
  Saturation1 : Saturate  UpperLimit=1.01  LowerLimit=0.1  OutDataType=fixdt(1, 16)  OutScaling=2^0
  Subsystem : Subsystem
  Subsystem1 : Subsystem
  Subsystem2 : Subsystem
  Subsystem3 : Subsystem
  Sum : Sum  Inputs=|++  OutDataType=fixdt(1, 16)  OutScaling=2^0
  Sum10 : Sum  Inputs=++|  OutDataType=fixdt(1, 16)  OutScaling=2^0
  Sum2 : Sum  Inputs=|++  OutDataType=fixdt(1, 16)  OutScaling=2^0
  Sum{3..4,7..8} (4 alike) : Sum  Inputs=|+-  OutDataType=fixdt(1, 16)  OutScaling=2^0
  Sum5 : Sum  Inputs=|++  OutDataType=fixdt(1, 16)  OutScaling=2^0
  Sum6 : Sum  Inputs=+|+|+  OutDataType=fixdt(1, 16)  OutScaling=2^0
  Sum9 : Sum  Inputs=|+-+  OutDataType=fixdt(1, 16)  OutScaling=2^0
  Switch : Switch  Threshold=200*0.3  OutDataType=fixdt(1, 16)  OutScaling=2^0
  Switch1 : Switch  Threshold=99.999999  OutDataType=fixdt(1, 16)  OutScaling=2^0
  Switch2 : Switch  Threshold=99.999999  OutDataType=fixdt(1, 16)  OutScaling=2^0
  Switch3 : Switch  OutDataType=fixdt(1, 16)  OutScaling=2^0
  Transfer Fcn1 : TransferFcn  Numerator=1  Denominator=[1/(10) 1]
  Transport Delay : TransportDelay  DelayTime=2
  Transport Delay1 : TransportDelay  DelayTime=2
  ain1 : Gain  Gain=0.25  ParameterDataType=fixdt(1, 16)  ParameterScaling=2^0  OutDataType=fixdt(1, 16)  OutScaling=2^0
  ain2 : Gain  Gain=1/700  ParameterDataType=fixdt(1, 16)  ParameterScaling=2^0  OutDataType=fixdt(1, 16)  OutScaling=2^0
  ain3 : Gain  Gain=1/16.5  ParameterDataType=fixdt(1, 16)  ParameterScaling=2^0  OutDataType=fixdt(1, 16)  OutScaling=2^0
  ain4 : Gain  Gain=700  ParameterDataType=fixdt(1, 16)  ParameterScaling=2^0  OutDataType=fixdt(1, 16)  OutScaling=2^0
  ain5 : Gain  Gain=0.75  ParameterDataType=fixdt(1, 16)  ParameterScaling=2^0  OutDataType=fixdt(1, 16)  OutScaling=2^0
  ain6 : Gain  Gain=16.5  ParameterDataType=fixdt(1, 16)  ParameterScaling=2^0  OutDataType=fixdt(1, 16)  OutScaling=2^0
  ain7 : Gain  Gain=0.03  ParameterDataType=fixdt(1, 16)  ParameterScaling=2^0  OutDataType=fixdt(1, 16)  OutScaling=2^0
  ain8 : Gain  Gain=7  ParameterDataType=fixdt(1, 16)  ParameterScaling=2^0  OutDataType=fixdt(1, 16)  OutScaling=2^0
  ain9 : Gain  Gain=0.3  ParameterDataType=fixdt(1, 16)  ParameterScaling=2^0  OutDataType=fixdt(1, 16)  OutScaling=2^0
  tag scope: Ibrefv8=global, boostv8=global, buckv8=global
  wires:
  Sum4/1 -> ain1/1, Subsystem2/1(In1)
  ain2/1 -> Saturation/1
  Subsystem2/1(Out1) -> Sum2/1
  ain1/1 -> Sum2/2
  Saturation/1 -> ain4/1, Switch1/3, Switch3/3, Switch3/2
  ain4/1 -> Sum3/1
  Sum3/1 -> ain3/1
  Subsystem1/1(Out1) -> Sum6/2
  ain5/1 -> Sum6/3
  Sum7/1 -> ain5/1, Subsystem1/1(In1)
  Sum2/1 -> Sum5/1
  Sum5/1 -> Sum8/1
  Sum8/1 -> ain6/1, Sum10/2
  Subsystem3/1(Out1) -> Sum/1
  ain6/1 -> Sum/2
  Sum/1 -> Sum9/1
  Sum9/1 -> Sum3/2, ain2/1
  ain3/1 -> Sum10/1
  ain7/1 -> Sum9/2
  Sum6/1 -> Sum4/1
  Sum10/1 -> Subsystem3/1(In1)
  [VcSUIMv8] -> Sum4/2
  [VcSUIMv8] -> Sum9/3
  [IbSUIMv8] -> Sum7/2
  [IbSUIMv8] -> Sum5/2
  [VbSUIMv8] -> Sum6/1
  [ISUIMv8] -> ain7/1
  [ISUIMv8] -> Sum8/2
  Subsystem/2(Out2) -> [boostv8]
  Subsystem/1(Out1) -> [buckv8]
  Transfer Fcn1/1 -> [Ibrefv8], Sum7/1
  [tv8] -> Subsystem/Enable
  [VbSUIMv8] -> Switch/2
  ain8/1 -> Switch/1
  ain9/1 -> Switch/3
  Ibref-v2/1 -> ain8/1, ain9/1
  Switch/1 -> Transfer Fcn1/1
  [VbSUIMv8] -> Add1/2
  Add1/1 -> Gain1/1, Gain2/1
  [VbSUIMv8] -> Switch2/3
  [socv8] -> Transport Delay1/1
  Transport Delay1/1 -> Switch2/2
  Add/1 -> Saturation1/1
  Gain1/1 -> Add/2
  Integrator/1 -> Add/1
  Gain2/1 -> Integrator/1
  Switch2/1 -> Add1/1, Memory/1
  Memory/1 -> Switch2/1
  Saturation1/1 -> Switch1/1
  Transport Delay/1 -> Switch1/2
  [socv8] -> Transport Delay/1
  Switch1/1 -> Switch3/1
  Switch3/1 -> Subsystem/1(In1)

== system allmodes/battery controller /v9 ==
  Ibref-v2 : Inport
  Add : Sum  OutDataType=fixdt(1, 16)  OutScaling=2^-10
  Add1 : Sum  Inputs=+-  OutDataType=fixdt(1, 16)  OutScaling=2^-10
  Gain1 : Gain  Gain=0.025  ParameterDataType=fixdt(1, 16)  ParameterScaling=2^0  OutDataType=fixdt(1, 16)  OutScaling=2^0
  Gain2 : Gain  Gain=0.8  ParameterDataType=fixdt(1, 16)  ParameterScaling=2^0  OutDataType=fixdt(1, 16)  OutScaling=2^0
  Integrator : Integrator
  Memory : Memory  X0=200
  Saturation : Saturate  UpperLimit=1  LowerLimit=-1  OutDataType=fixdt(1, 16)  OutScaling=2^0
  Saturation1 : Saturate  UpperLimit=1.01  LowerLimit=0.1  OutDataType=fixdt(1, 16)  OutScaling=2^0
  Subsystem : Subsystem
  Subsystem1 : Subsystem
  Subsystem2 : Subsystem
  Subsystem3 : Subsystem
  Sum : Sum  Inputs=|++  OutDataType=fixdt(1, 16)  OutScaling=2^0
  Sum10 : Sum  Inputs=++|  OutDataType=fixdt(1, 16)  OutScaling=2^0
  Sum2 : Sum  Inputs=|++  OutDataType=fixdt(1, 16)  OutScaling=2^0
  Sum{3..4,7..8} (4 alike) : Sum  Inputs=|+-  OutDataType=fixdt(1, 16)  OutScaling=2^0
  Sum5 : Sum  Inputs=|++  OutDataType=fixdt(1, 16)  OutScaling=2^0
  Sum6 : Sum  Inputs=+|+|+  OutDataType=fixdt(1, 16)  OutScaling=2^0
  Sum9 : Sum  Inputs=|+-+  OutDataType=fixdt(1, 16)  OutScaling=2^0
  Switch : Switch  Threshold=200*0.3  OutDataType=fixdt(1, 16)  OutScaling=2^0
  Switch1 : Switch  Threshold=99.999999  OutDataType=fixdt(1, 16)  OutScaling=2^0
  Switch2 : Switch  Threshold=99.999999  OutDataType=fixdt(1, 16)  OutScaling=2^0
  Switch3 : Switch  OutDataType=fixdt(1, 16)  OutScaling=2^0
  Transfer Fcn1 : TransferFcn  Numerator=1  Denominator=[1/(10) 1]
  Transport Delay : TransportDelay  DelayTime=2
  Transport Delay1 : TransportDelay  DelayTime=2
  ain1 : Gain  Gain=0.25  ParameterDataType=fixdt(1, 16)  ParameterScaling=2^0  OutDataType=fixdt(1, 16)  OutScaling=2^0
  ain2 : Gain  Gain=1/700  ParameterDataType=fixdt(1, 16)  ParameterScaling=2^0  OutDataType=fixdt(1, 16)  OutScaling=2^0
  ain3 : Gain  Gain=1/16.5  ParameterDataType=fixdt(1, 16)  ParameterScaling=2^0  OutDataType=fixdt(1, 16)  OutScaling=2^0
  ain4 : Gain  Gain=700  ParameterDataType=fixdt(1, 16)  ParameterScaling=2^0  OutDataType=fixdt(1, 16)  OutScaling=2^0
  ain5 : Gain  Gain=0.75  ParameterDataType=fixdt(1, 16)  ParameterScaling=2^0  OutDataType=fixdt(1, 16)  OutScaling=2^0
  ain6 : Gain  Gain=16.5  ParameterDataType=fixdt(1, 16)  ParameterScaling=2^0  OutDataType=fixdt(1, 16)  OutScaling=2^0
  ain7 : Gain  Gain=0.03  ParameterDataType=fixdt(1, 16)  ParameterScaling=2^0  OutDataType=fixdt(1, 16)  OutScaling=2^0
  ain8 : Gain  Gain=7  ParameterDataType=fixdt(1, 16)  ParameterScaling=2^0  OutDataType=fixdt(1, 16)  OutScaling=2^0
  ain9 : Gain  Gain=0.3  ParameterDataType=fixdt(1, 16)  ParameterScaling=2^0  OutDataType=fixdt(1, 16)  OutScaling=2^0
  tag scope: Ibrefv9=global, boostv9=global, buckv9=global
  wires:
  [socv9] -> Transport Delay/1
  Transport Delay/1 -> Switch1/2
  Saturation1/1 -> Switch1/1
  Memory/1 -> Switch2/1
  Switch2/1 -> Memory/1, Add1/1
  Gain2/1 -> Integrator/1
  Integrator/1 -> Add/1
  Gain1/1 -> Add/2
  Add/1 -> Saturation1/1
  Transport Delay1/1 -> Switch2/2
  [socv9] -> Transport Delay1/1
  [VbSUIMv9] -> Switch2/3
  Add1/1 -> Gain2/1, Gain1/1
  [VbSUIMv9] -> Add1/2
  Switch/1 -> Transfer Fcn1/1
  Ibref-v2/1 -> ain9/1, ain8/1
  ain9/1 -> Switch/3
  ain8/1 -> Switch/1
  [VbSUIMv9] -> Switch/2
  [tv9] -> Subsystem/Enable
  Transfer Fcn1/1 -> Sum7/1, [Ibrefv9]
  Subsystem/1(Out1) -> [buckv9]
  Subsystem/2(Out2) -> [boostv9]
  [ISUIMv9] -> Sum8/2
  [ISUIMv9] -> ain7/1
  [VbSUIMv9] -> Sum6/1
  [IbSUIMv9] -> Sum5/2
  [IbSUIMv9] -> Sum7/2
  [VcSUIMv9] -> Sum9/3
  [VcSUIMv9] -> Sum4/2
  Sum10/1 -> Subsystem3/1(In1)
  Sum6/1 -> Sum4/1
  ain7/1 -> Sum9/2
  ain3/1 -> Sum10/1
  Sum9/1 -> ain2/1, Sum3/2
  Sum/1 -> Sum9/1
  ain6/1 -> Sum/2
  Subsystem3/1(Out1) -> Sum/1
  Sum8/1 -> Sum10/2, ain6/1
  Sum5/1 -> Sum8/1
  Sum2/1 -> Sum5/1
  Sum7/1 -> Subsystem1/1(In1), ain5/1
  ain5/1 -> Sum6/3
  Subsystem1/1(Out1) -> Sum6/2
  Sum3/1 -> ain3/1
  ain4/1 -> Sum3/1
  Saturation/1 -> ain4/1, Switch1/3, Switch3/3, Switch3/2
  ain1/1 -> Sum2/2
  Subsystem2/1(Out1) -> Sum2/1
  ain2/1 -> Saturation/1
  Sum4/1 -> Subsystem2/1(In1), ain1/1
  Switch1/1 -> Switch3/1
  Switch3/1 -> Subsystem/1(In1)
